simulink model "expbook"  (R2022a)
settings: Solver=VariableStepAuto  StartTime=0.0  StopTime=50  RelTol=1e-3
values from neighbouring files (symbols this model uses):
  Ce = 0.556    [Untitled.m]    (also in liner.m)
  Ki = 5    [Untitled.m]    (also in liner.m = 1)
  Kn = 7.84    [Untitled.m]    (also in liner.m = 29.75)
  Ks = 1    [Untitled.m]    (also in liner.m)
  ned = 5    [liner.m]
  R = 0.6    [Untitled.m]    (also in liner.m)
  Tl = 0.167    [Untitled.m]    (also in liner.m)
  Tm = 0.282    [Untitled.m]    (also in liner.m)
  Ts = 0.01    [Untitled.m]    (also in liner.m)
undefined symbols (not defined in the file or in its folder): alpha, beta, lambda, tau_i, tau_n, Ued
settings Model: Creator=houtonglei  LastModifiedBy=houtonglei
settings DataIOCC: ExternalInput=[Ki Kn tau_i tau_n]
settings DebuggingCC: UnconnectedInputMsg=warning  UnconnectedOutputMsg=warning  UnconnectedLineMsg=warning
settings ModelReferenceCC: EnableParallelModelReferenceBuilds=on
settings RTWCC: DLArmComputeVersion=19.05

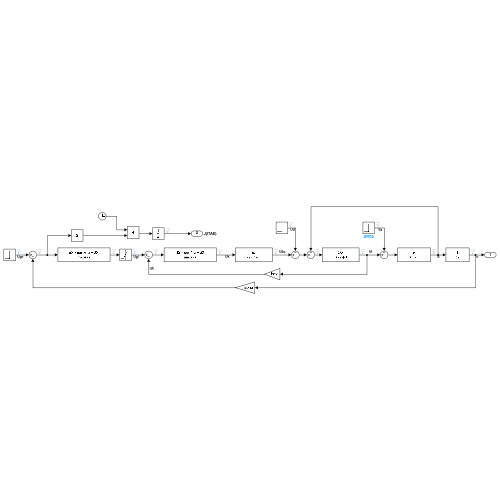
[thumbnail: Simulink's stored preview of the top-level diagram]
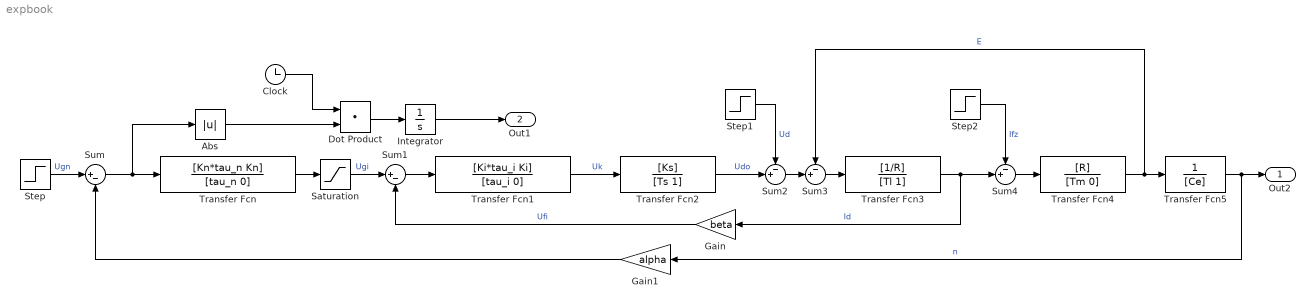
== system expbook ==
  Abs : Abs  SaturateOnIntegerOverflow=off
  Clock : Clock
  Dot Product : DotProduct  OutDataTypeStr=Inherit: Inherit via internal rule
  Gain : Gain  Gain=beta
  Gain1 : Gain  Gain=alpha
  Integrator : Integrator
  Saturation : Saturate  UpperLimit=lambda*Ued  LowerLimit=-lambda*Ued
  Step : Step  Time=0  After=ned  SampleTime=0
  Step1 : Step  After=0  SampleTime=0
  Step2 : Step  After=0  SampleTime=0
  Sum : Sum  Inputs=|+-
  Sum1 : Sum  Inputs=|+-
  Sum2 : Sum  Inputs=-+|
  Sum3 : Sum  Inputs=-+|
  Sum4 : Sum  Inputs=-+|
  Transfer Fcn : TransferFcn  Numerator=[Kn*tau_n Kn]  Denominator=[tau_n 0]  ContinuousStateAttributes='ASR'
  Transfer Fcn1 : TransferFcn  Numerator=[Ki*tau_i Ki]  Denominator=[tau_i 0]  ContinuousStateAttributes='ACR'
  Transfer Fcn2 : TransferFcn  Numerator=[Ks]  Denominator=[Ts 1]  ContinuousStateAttributes='PWM'
  Transfer Fcn3 : TransferFcn  Numerator=[1/R]  Denominator=[Tl 1]
  Transfer Fcn4 : TransferFcn  Numerator=[R]  Denominator=[Tm 0]
  Transfer Fcn5 : TransferFcn  Denominator=[Ce]
  Out2 : Outport
  Out1 : Outport  Port=2  SignalName=J(ITAE)
  wires:
  Transfer Fcn3/1 -> Sum4/2, Gain/1  "Id"
  Sum/1 -> Abs/1, Transfer Fcn/1
  Transfer Fcn/1 -> Saturation/1
  Saturation/1 -> Sum1/1  "Ugi"
  Gain/1 -> Sum1/2  "Ufi"
  Gain1/1 -> Sum/2
  Sum1/1 -> Transfer Fcn1/1
  Transfer Fcn1/1 -> Transfer Fcn2/1  "Uk"
  Transfer Fcn2/1 -> Sum2/2  "Udo"
  Sum2/1 -> Sum3/2
  Sum3/1 -> Transfer Fcn3/1
  Sum4/1 -> Transfer Fcn4/1
  Transfer Fcn4/1 -> Transfer Fcn5/1, Sum3/1  "E"
  Transfer Fcn5/1 -> Out2/1, Gain1/1  "n"
  Step/1 -> Sum/1  "Ugn"
  Step1/1 -> Sum2/1  "Ud"
  Step2/1 -> Sum4/1  "Ifz"
  Abs/1 -> Dot Product/2
  Clock/1 -> Dot Product/1
  Dot Product/1 -> Integrator/1
  Integrator/1 -> Out1/1
